simulink model "LH2Ship_Simulink_Summer"  (R2025a)
settings: Solver=VariableStepAuto  StartTime=0.0  StopTime=3600*24*7  FixedStep=0.1  MaxStep=0.5  MinStep=0.001  RelTol=1e-7  AbsTol=1e-7
values from neighbouring files (symbols this model uses):
  BoilerEff = 0.85    [PEMFC_Model.m]
  H2Consumption_kg = H2SupplyMolRate(:,1:iPmaxtot).*H2_kg_mol    [PEMFC_Model.m]
  H2Exhaust_kg = H2ExhaustMolRate(:,1:iPmaxtot).*H2_kg_mol    [PEMFC_Model.m]
  H2hhv = 141.7*10^6    (= 141700000)    [PEMFC_Model.m]
  H2lhv = 119.96*10^6    (= 119960000)    [PEMFC_Model.m]
  H2u = (0.05:0.1:0.95)    [PEMFC_Model.m]
  HeatStorageCapacity = 4.5e10    (= 45000000000)    [PEMFC_Model.m]
  HeatStorageEff = 0.9    [PEMFC_Model.m]
  HeatStorageIC = 1    [PEMFC_Model.m]
  i_FC = iCell(1,1:iPmaxtot)    [PEMFC_Model.m]
  Nstacks = 330    [PEMFC_Model.m]
  PowerElectronicsEff = 0.9    [PEMFC_Model.m]
  RecoveredHeat = NetHeatOut(:,1:iPmaxtot)    [PEMFC_Model.m]
  V_FC = Vout(:,1:iPmaxtot)    [PEMFC_Model.m]
undefined symbols (not defined in the file or in its folder): BatteryCapacity, BattInitialSOC, LH2ColdRecovery_Efficiency, LH2ColdRecovery_EnthalpyGain, mass, Rt, v, VDCBus
libraries: fl_lib x16, nesl_utility x15, simulink x5, slpidlib x2, batteryecm_lib x1, ee_lib x1
(part 1 of 2)
settings Model: Creator=age  LastModifiedBy=alber
settings SolverCC: InitialStep=0.001  MaxConsecutiveMinStep=2  ZeroCrossControl=DisableAll  AlgebraicLoopSolver=TrustRegion
settings DataIOCC: LimitDataPoints=on  MaxDataPoints=10000  ReturnWorkspaceOutputs=off
settings OptimizationCC: LifeSpan=inf
settings DebuggingCC: UnconnectedInputMsg=warning  UnconnectedOutputMsg=warning  UnconnectedLineMsg=warning  AllowSymbolicDim=off  SFUnexpectedBacktrackingDiag=warning  SFNoUnconditionalDefaultTransitionDiag=warning  SFExecutionAtInitializationDiag=none  ArithmeticOperatorsInVariantConditions=warning
settings ModelReferenceCC: EnableRefExpFcnMdlSchedulingChecks=on
settings SFSimCC: SimUseLocalCustomCode=off  CustomCodeUndefinedFunction=UseInterfaceOnly
settings RTWCC: RTWUseLocalCustomCode=off  GPUComputeCapability=3.5
settings CodeAppCC: StateflowObjectComments=on
settings GRTTargetCC: TargetLangStandard=C89/C90 (ANSI)
settings ConfigComp: CovMetricSettings=dw  CovSaveCumulativeToWorkspaceVar=on  CovSaveSingleToWorkspaceVar=on  CovExternalEMLEnable=off  CovSFcnEnable=off
settings SimscapeCC: SimscapeLogLimitData=off  SimscapeLogDataHistory=10000.0

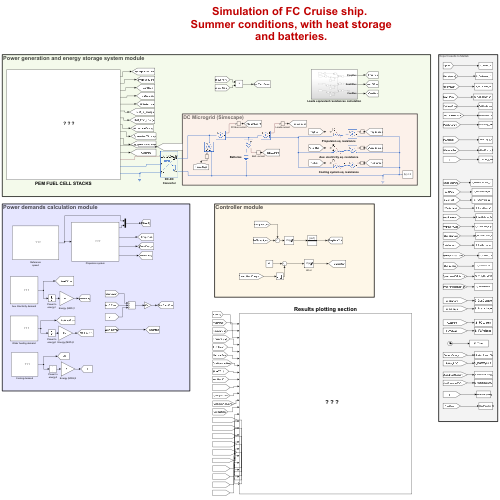
[thumbnail: Simulink's stored preview of the top-level diagram]
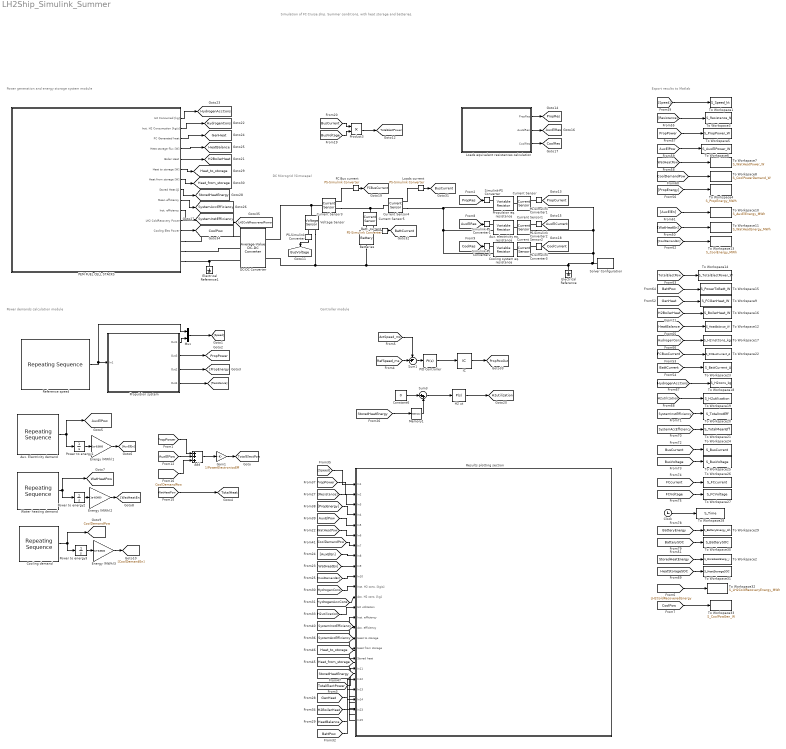
== system LH2Ship_Simulink_Summer ==
  note: Power demands calculation module
  note: Export results to Matlab
  note: Simulation of FC Cruise ship.
      | Summer conditions, with heat storage and batteries.
  note: Power generation and energy storage system module
  note: DC Microgrid (Simscape)
  note: Controller module
  Add : Sum  Inputs=+++
  Aux. Electricity demand : simulink/Sources/Repeating Sequence  rep_seq_t=AuxElectProfile.t  rep_seq_y=AuxElectProfile.Elect  mask(Repeating table){}
      mask Display: image('Aux electricity summer_icon.JPG');
  Aux. electricity eq. resistance : fl_lib/Electrical/Electrical Elements/Variable Resistor  Rmin=2.8571e-4 Ohm  thermalEnable=false  thermal_mass=1 J/K  i_specify=off  i_priority=None  i=0 A  i_nominal_specify=off  i_nominal_value=1  i_nominal_unit=A  v_specify=off  v_priority=None  v=0 V  v_nominal_specify=off  v_nominal_value=1  v_nominal_unit=V  T_specify=off  T_priority=None  T=300 K  T_nominal_specify=off  T_nominal_value=1  T_nominal_unit=K
  Batt. current : nesl_utility/PS-Simulink Converter  PhysicalDomain=network_engine_domain  SubClassName=ps_output  LeftPortType=input  RightPortType=output  PseudoPeriodic=off  Frequencies=[]  VectorFormat=1-D array  Unit=1  AffineConversion=off
  Batteries : batteryecm_lib/Battery  Vnom=100 V  prm_dir=simscape.enum.battery.prm_dir.disabled  R1_dis=2 Ohm  R1_ch=2 Ohm  R1=0.00016667 Ohm  prm_AH=1  AH=6000 hr*A  V1=75 V  AH1=5426.087 hr*A  prm_R2=1  R2=2000 Ohm  Tmeas=298.15 K  charge_measurement_port=simscape.enum.battery.enable.no  prm_dyn=1  Rp1=0.0005 Ohm  tau1=10 s  Rp2=0.005 Ohm  tau2=30 s  Rp3=0.005 Ohm  tau3=30 s  Rp4=0.005 Ohm  tau4=30 s  Rp5=0.005 Ohm  tau5=30 s  prm_fade=1  N_fade=100  AH_fade=45 hr*A  R1_fade=2.02 Ohm  R1_ch_fade=2.02 Ohm  V1_fade=10.35 V  prm_age=simscape.enum.battery.prm_age.disabled  prm_age_OCV=simscape.enum.battery.prm_age_OCV.OCV  OCV_age=0.9  SOC_age=60  Tmeas_age=298.15 K  delta_time_age_vec=[0] d  temperature_age_vec=[273] K  OCV_scaling_age=2.2134e6  OCV_offset_age=1.632e6  temp_exp_age=0.515833569 V  t_exp_age=0.75  Vnom_T2=12 V  R1_T2=2.2 Ohm  R1_T2_dis=2.2 Ohm  R1_T2_ch=2.2 Ohm  V1_T2=11.4 V  R2_T2=2200 Ohm  Rp1_T2=0.005 Ohm  tau1_T2=30 s  Rp2_T2=0.005 Ohm  tau2_T2=30 s  Rp3_T2=0.005 Ohm  tau3_T2=30 s  Rp4_T2=0.005 Ohm  tau4_T2=30 s  Rp5_T2=0.005 Ohm  tau5_T2=30 s  Tmeas2=273.15 K  thermal_port=simscape.enum.thermaleffects.omit  thermal_mass=30000 J/K  i_specify=on  i_priority=Low  i=0 A  i_nominal_specify=off  i_nominal_value=1  i_nominal_unit=A  v_specify=on  v_priority=None  v=100 V  v_nominal_specify=off  v_nominal_value=1  v_nominal_unit=V  charge_specify=on  charge_priority=High  charge=3000 hr*A  charge_nominal_specify=off  charge_nominal_value=1  charge_nominal_unit=hr*A  num_cycles_specify=on  num_cycles_priority=None  num_cycles=0  num_cycles_nominal_specify=off  num_cycles_nominal_value=1  num_cycles_nominal_unit=1  temperature_specify=off  temperature_priority=High  temperature=298.15 K  temperature_nominal_specify=off  temperature_nominal_value=1  temperature_nominal_unit=K
  Clock : Clock
  Constant6 : Constant  Value=0
  Cooling demand : simulink/Sources/Repeating Sequence  rep_seq_t=SpaceCoolingProfile_Summer.t  rep_seq_y=SpaceCoolingProfile_Summer.Cooling  mask(Repeating table){}
      mask Display: image('Cooling demand summer_icon.JPG');
  Cooling system eq. resistance : fl_lib/Electrical/Electrical Elements/Variable Resistor  Rmin=2.8571e-4 Ohm  thermalEnable=false  thermal_mass=1 J/K  i_specify=off  i_priority=None  i=0 A  i_nominal_specify=off  i_nominal_value=1  i_nominal_unit=A  v_specify=off  v_priority=None  v=0 V  v_nominal_specify=off  v_nominal_value=1  v_nominal_unit=V  T_specify=off  T_priority=None  T=300 K  T_nominal_specify=off  T_nominal_value=1  T_nominal_unit=K
  Current Sensor{,1..5} (6 alike) : fl_lib/Electrical/Electrical Sensors/Current Sensor
  DC-DC Converter : ee_lib/Semiconductors & Converters/Converters/Average-Value DC-DC Converter  implementation_option=ee.enum.converters.implementation.behavioral  converter_type=3  control_option=ee.enum.converters.controlinput.dutycycle  efficiency_option=ee.enum.converters.efficiency.constant  efficiency_fixed=100  i_vec=[0, 2, 5] A  efficiency_vec=[90, 95, 98]  Lf=1e-6 H  Rl=0 Ohm  Cf=1e-7 F  Rc=1e-6 Ohm  iL_specify=off  iL_priority=High  iL=0 A  iL_nominal_specify=off  iL_nominal_value=1  iL_nominal_unit=A  vc_specify=off  vc_priority=High  vc=0 V  vc_nominal_specify=off  vc_nominal_value=1  vc_nominal_unit=V
      settings: InternalSimscapePortConfiguration="{\"Bottom\":[],\"Left\":[{\"id\":\"DutyCycle\",\"label\":\"DutyCycle\",\"type\":\"input\"},{\"id\":\"p1\",\"label\":\"1+\",\"type\":\"foundation.electrical.electrical\"},{\"id\":\"n1\",\"label\":\"1-\",\"type\":\"foundation.electrical.electrical\"}],\"Right\":[{\"id\":\"p2\",\"label\":\"2+\",\"type\":\"foundation.electrical.electrical\"},{\"id\":\"n2\",\"label\":\"2-\",\"type\":\"foundation.electrical.electrical\"}],\"Top\":[]}"
  Electrical Reference : fl_lib/Electrical/Electrical Elements/Electrical Reference
  Electrical Reference1 : fl_lib/Electrical/Electrical Elements/Electrical Reference
  Energy (MWh)1 : Gain  Gain=1e-6/3600
  Energy (MWh)2 : Gain  Gain=1e-6/3600
  Energy (MWh)3 : Gain  Gain=1e-6/3600
  FC Bus current : nesl_utility/PS-Simulink Converter  PhysicalDomain=network_engine_domain  SubClassName=ps_output  LeftPortType=input  RightPortType=output  PseudoPeriodic=off  Frequencies=[]  VectorFormat=1-D array  Unit=1  AffineConversion=off
  Gain1 : Gain  Gain=1/PowerElectronicsEff
  H2 ut : slpidlib/PID Controller  Controller=P  Form=Parallel  TimeDomain=Continuous-time  UseExternalTs=off  SampleTime=-1  IntegratorMethod=Forward Euler  FilterMethod=Forward Euler  ControllerParametersSource=internal  P=2.73467181561609e-9  I=5.74544625203428e-08  UseKiTs=off  D=7000000  UseExternalDerivativeSource=off  N=0.01  UseFilter=on  TunerSelectOption=Transfer Function Based (PID Tuner App)  ZeroCross=off  InitialConditionSource=internal  InitialConditionForIntegrator=0.95  InitialConditionForFilter=0.1  DifferentiatorICPrevScaledInput=0  ExternalReset=none  TrackingMode=off  Kt=1  LimitOutput=on  SatLimitsSource=internal  UpperSaturationLimit=0.95  LowerSaturationLimit=0.05  LinearizeAsGain=off  AntiWindupMode=clamping  Kb=1  LimitIntegrator=off  UpperIntegratorSaturationLimit=inf  LowerIntegratorSaturationLimit=-inf  POutMin=[]  POutMax=[]  IOutMin=[]  IOutMax=[]  DOutMin=[]  DOutMax=[]  NOutMin=[]  NOutMax=[]  SumOutMin=[]  SumOutMax=[]  SaturationOutMin=[]  SaturationOutMax=[]  PParamMin=[]  PParamMax=[]  IParamMin=[]  IParamMax=[]  DParamMin=[]  DParamMax=[]  NParamMin=[]  NParamMax=[]  KbParamMin=[]  KbParamMax=[]  KtParamMin=[]  KtParamMax=[]  KbOutMin=[]  KbOutMax=[]  KtOutMin=[]  KtOutMax=[]  IntegratorOutMin=[]  IntegratorOutMax=[]  FilterOutMin=[]  FilterOutMax=[]  SumI1OutMin=[]  SumI1OutMax=[]  SumI2OutMin=[]  SumI2OutMax=[]  SumI3OutMin=[]  SumI3OutMax=[]  SumI4OutMin=[]  SumI4OutMax=[]  SumDOutMin=[]  SumDOutMax=[]  DifferentiatorOutMin=[]  DifferentiatorOutMax=[]  FilterDiffOutCoefMin=[]  FilterDiffOutCoefMax=[]  ReciprocalOutMin=[]  ReciprocalOutMax=[]  SumDenOutMin=[]  SumDenOutMax=[]  SumNumOutMin=[]  SumNumOutMax=[]  DivideOutMin=[]  DivideOutMax=[]  UdiffTsProdOutMin=[]  UdiffTsProdOutMax=[]  NTsProdOutMin=[]  NTsProdOutMax=[]  UintegralTsProdOutMin=[]  UintegralTsProdOutMax=[]  UngainTsProdOutMin=[]  UngainTsProdOutMax=[]  ClampingZeroOutDataTypeStr=Inherit: Inherit via back propagation  ClampingZeroOutMin=[]  ClampingZeroOutMax=[]  FilterDenConstantOutDataTypeStr=Inherit: Inherit via back propagation  FilterDenConstantOutMin=[]  FilterDenConstantOutMax=[]  PCopyOutDataTypeStr=Inherit: Inherit via back propagation  PCopyOutMin=[]  PCopyOutMax=[]  NCopyOutDataTypeStr=Inherit: Inherit via back propagation  NCopyOutMin=[]  NCopyOutMax=[]  IntegratorContinuousStateAttributes=''  IntegratorStateMustResolveToSignalObject=off  IntegratorRTWStateStorageClass=Auto  FilterContinuousStateAttributes=''  FilterStateMustResolveToSignalObject=off  FilterRTWStateStorageClass=Auto  ParallelPVariant=InternalParameters  IdealPVariant=Disabled  IVariant=Disabled  DVariant=Disabled  IntegratorVariant=Disabled  SatVariant=Enabled  AWVariant=Disabled  PCopyVariant=Disabled  TRVariant=Disabled  FdbkBlocksVariant=Forward  IdealPFdbkVariant=Disabled  SatFdbkVariant=Disabled  DerivativeFilterVariant=Disabled  NVariant=Disabled  NCopyVariant=Disabled_SignalSpec  FilterICVariant=Disabled  IntegratorICVariant=Disabled  ExternalResetVariant=Disabled  TRSumVariant=Passthrough  SumFdbkVariant=Disabled  SumVariant=Passthrough_P  TsampFilterVariant=InternalTs  TsampNgainVariant=Passthrough  TsampIntegralVariant=Disabled_SignalSpec  ExternalSaturationOutDataTypeStr=Inherit: Same as second input  DerivativeSourceVariant=Disabled  PreIntVariant=InternalPreInt
  IC : InitialCondition  Value=2e7
  Loads current : nesl_utility/PS-Simulink Converter  PhysicalDomain=network_engine_domain  SubClassName=ps_output  LeftPortType=input  RightPortType=output  PseudoPeriodic=off  Frequencies=[]  VectorFormat=1-D array  Unit=1  AffineConversion=off
  Loads equivalent resistances calculation : Subsystem
  Memory1 : Memory  InitialCondition=HeatStorageIC*HeatStorageCapacity
  Mux : Mux  Inputs=2
  PEM FUEL CELL STACKS : Subsystem
      mask Display: image('Fuel cell_PEM_icon.JPG');
  PID Controller : slpidlib/PID Controller  Controller=PI  Form=Parallel  TimeDomain=Continuous-time  UseExternalTs=off  SampleTime=-1  IntegratorMethod=Forward Euler  FilterMethod=Forward Euler  ControllerParametersSource=internal  P=9967066.66982428  I=15836.3521855852  UseKiTs=off  D=676782585.714132  UseExternalDerivativeSource=off  N=0.00702265439594147  UseFilter=on  TunerSelectOption=Transfer Function Based (PID Tuner App)  InitialConditionSource=internal  InitialConditionForIntegrator=2e7  InitialConditionForFilter=0  DifferentiatorICPrevScaledInput=0  ExternalReset=none  TrackingMode=off  Kt=1  LimitOutput=on  SatLimitsSource=internal  UpperSaturationLimit=60000000  LowerSaturationLimit=-60000000  LinearizeAsGain=off  AntiWindupMode=clamping  Kb=1  LimitIntegrator=off  UpperIntegratorSaturationLimit=inf  LowerIntegratorSaturationLimit=-inf  POutMin=[]  POutMax=[]  IOutMin=[]  IOutMax=[]  DOutMin=[]  DOutMax=[]  NOutMin=[]  NOutMax=[]  SumOutMin=[]  SumOutMax=[]  SaturationOutMin=[]  SaturationOutMax=[]  PParamMin=[]  PParamMax=[]  IParamMin=[]  IParamMax=[]  DParamMin=[]  DParamMax=[]  NParamMin=[]  NParamMax=[]  KbParamMin=[]  KbParamMax=[]  KtParamMin=[]  KtParamMax=[]  KbOutMin=[]  KbOutMax=[]  KtOutMin=[]  KtOutMax=[]  IntegratorOutMin=[]  IntegratorOutMax=[]  FilterOutMin=[]  FilterOutMax=[]  SumI1OutMin=[]  SumI1OutMax=[]  SumI2OutMin=[]  SumI2OutMax=[]  SumI3OutMin=[]  SumI3OutMax=[]  SumI4OutMin=[]  SumI4OutMax=[]  SumDOutMin=[]  SumDOutMax=[]  DifferentiatorOutMin=[]  DifferentiatorOutMax=[]  FilterDiffOutCoefMin=[]  FilterDiffOutCoefMax=[]  ReciprocalOutMin=[]  ReciprocalOutMax=[]  SumDenOutMin=[]  SumDenOutMax=[]  SumNumOutMin=[]  SumNumOutMax=[]  DivideOutMin=[]  DivideOutMax=[]  UdiffTsProdOutMin=[]  UdiffTsProdOutMax=[]  NTsProdOutMin=[]  NTsProdOutMax=[]  UintegralTsProdOutMin=[]  UintegralTsProdOutMax=[]  UngainTsProdOutMin=[]  UngainTsProdOutMax=[]  ClampingZeroOutDataTypeStr=Inherit: Inherit via back propagation  ClampingZeroOutMin=[]  ClampingZeroOutMax=[]  FilterDenConstantOutDataTypeStr=Inherit: Inherit via back propagation  FilterDenConstantOutMin=[]  FilterDenConstantOutMax=[]  PCopyOutDataTypeStr=Inherit: Inherit via back propagation  PCopyOutMin=[]  PCopyOutMax=[]  NCopyOutDataTypeStr=Inherit: Inherit via back propagation  NCopyOutMin=[]  NCopyOutMax=[]  IntegratorContinuousStateAttributes=''  IntegratorStateMustResolveToSignalObject=off  IntegratorRTWStateStorageClass=Auto  FilterContinuousStateAttributes=''  FilterStateMustResolveToSignalObject=off  FilterRTWStateStorageClass=Auto  ParallelPVariant=InternalParameters  IdealPVariant=Disabled  IVariant=InternalParameters  DVariant=Disabled  IntegratorVariant=Continuous  SatVariant=Enabled  AWVariant=ContClampingParallel  PCopyVariant=Disabled  TRVariant=Disabled  FdbkBlocksVariant=Forward  IdealPFdbkVariant=Disabled  SatFdbkVariant=Disabled  DerivativeFilterVariant=Disabled  NVariant=Disabled  NCopyVariant=Disabled_SignalSpec  FilterICVariant=Disabled  IntegratorICVariant=InternalICs  ExternalResetVariant=Disabled  TRSumVariant=Passthrough  SumFdbkVariant=Disabled  SumVariant=Sum_PI  TsampFilterVariant=InternalTs  TsampNgainVariant=Passthrough  TsampIntegralVariant=Disabled_SignalSpec  ExternalSaturationOutDataTypeStr=Inherit: Same as second input  DerivativeSourceVariant=Disabled  PreIntVariant=InternalPreInt
  PS-Simulink Converter{,1..3} (4 alike) : nesl_utility/PS-Simulink Converter  PhysicalDomain=network_engine_domain  SubClassName=ps_output  LeftPortType=input  RightPortType=output  PseudoPeriodic=off  Frequencies=[]  VectorFormat=1-D array  Unit=1  AffineConversion=off
  Power to energy1 : Integrator  LowerSaturationLimit=0
  Power to energy2 : Integrator  LowerSaturationLimit=0
  Power to energy3 : Integrator  LowerSaturationLimit=0
  Product3 : Product
  Propulsion eq. resistance : fl_lib/Electrical/Electrical Elements/Variable Resistor  Rmin=2.8571e-4 Ohm  thermalEnable=false  thermal_mass=1 J/K  i_specify=off  i_priority=None  i=0 A  i_nominal_specify=off  i_nominal_value=1  i_nominal_unit=A  v_specify=off  v_priority=None  v=0 V  v_nominal_specify=off  v_nominal_value=1  v_nominal_unit=V  T_specify=off  T_priority=None  T=300 K  T_nominal_specify=off  T_nominal_value=1  T_nominal_unit=K
  Propulsion system : Subsystem
      mask Display: image('Propusion engine.jpg');
  Reference speed : simulink/Sources/Repeating Sequence  rep_seq_t=SpeedProfile.Time  rep_seq_y=SpeedProfile.Speed  mask(Repeating table){}
      mask Display: image('RefSpeed_icon.PNG');
  Results plotting section : Subsystem
      mask Display: image('222-2224981_data-visualization-icon-circle.png.jpg');
  Simulink-PS Converter : nesl_utility/Simulink-PS Converter  PhysicalDomain=network_engine_domain  SubClassName=ps_input  LeftPortType=input  RightPortType=output  PseudoPeriodic=off  Frequencies=[]  NoiseDistribution=none  NoiseParameters=[]  Unit=1  AffineConversion=off  FilteringAndDerivatives=provide  SimscapeFilterOrder=1  InputFilterTimeConstant=0.001  UdotUserProvided=0
  Simulink-PS Converter1 : nesl_utility/Simulink-PS Converter  PhysicalDomain=network_engine_domain  SubClassName=ps_input  LeftPortType=input  RightPortType=output  PseudoPeriodic=off  Frequencies=[]  NoiseDistribution=none  NoiseParameters=[]  Unit=1  AffineConversion=off  FilteringAndDerivatives=provide  SimscapeFilterOrder=1  InputFilterTimeConstant=0.001  UdotUserProvided=0
  Simulink-PS Converter2 : nesl_utility/Simulink-PS Converter  PhysicalDomain=network_engine_domain  SubClassName=ps_input  LeftPortType=input  RightPortType=output  PseudoPeriodic=off  Frequencies=[]  NoiseDistribution=none  NoiseParameters=[]  Unit=1  AffineConversion=off  FilteringAndDerivatives=provide  SimscapeFilterOrder=1  InputFilterTimeConstant=0.001  UdotUserProvided=0
  Solver Configuration : nesl_utility/Solver Configuration  PhysicalDomain=network_engine_domain  SubClassName=solver  LeftPortType=input  RightPortType=generic  Tones=[]  Harmonics=[]  SimulateNoise=off  Profile=off  UseLocalSampling=off  EnableSwitchedLinearOptims=on  FrequencyDomain=off  UseCCode=off  RelTol=0.001  AbsTol=1e-06  MinStep=1e-09  ToWorkspace=off  RevertToSquareIcSolve=off  NumHomotopyIterations=100  PhasorMode=off  PhasorModeNumHarmonics=1  ConsistencySolver=NEWTON_FTOL  IndexReductionMethod=DerivativeReplacement  DoDC=on  ResidualTolerance=1e-09  ConsistencyTolSource=GLOBAL  ConsistencyAbsTol=0.001  ConsistencyRelTol=0.001  ConsistencyTolFactor=0.001  UseLocalSolver=off  LocalSolverChoice=NE_BACKWARD_EULER_ADVANCER  ResolveIndetEquations=on  FunctionEvalNumThread=1  LocalSolverSampleTime=0.001  DoFixedCost=off  MaxNonlinIter=3  MaxModeIter=2  ComputeImpulses=off  ImpulseIterations=2  LinearAlgebra=auto  LinearAlgebraNumThread=0  EquationFormulation=NE_TIME_EF  DelaysMemoryBudget=1024  AutomaticFiltering=on  FilteringTimeConstant=0.001  PartitionStorageMethod=AS_NEEDED  PartitionMemoryBudget=1024  PartitionMethod=FAST  MultibodyUseLocalSolver=off  MultibodyLocalSolverChoice=ODE1  MultibodyLocalSolverSampleTime=0.001
  Sum1 : Sum  Inputs=-+|
  Sum3 : Sum  Inputs=|++
  To Workspace1 : ToWorkspace  VariableName=S_Speed_kt  SampleTime=30
  To Workspace10 : ToWorkspace  VariableName=S_AuxElEnergy_MWh  SampleTime=30
  To Workspace11 : ToWorkspace  VariableName=S_WatHeatEnergy_MWh  SampleTime=30
  To Workspace12 : ToWorkspace  VariableName=S_HeatBalance_W  SampleTime=30
  To Workspace13 : ToWorkspace  VariableName=S_CoolEnergy_MWh  SampleTime=30
  To Workspace14 : ToWorkspace  VariableName=S_TotalElectPower_W  SampleTime=30
  To Workspace15 : ToWorkspace  VariableName=S_PowerToBatt_W  SampleTime=30
  To Workspace16 : ToWorkspace  VariableName=S_BoilerHeat_W  SampleTime=30
  To Workspace17 : ToWorkspace  VariableName=S_H2instCons_kgs  SampleTime=30
  To Workspace18 : ToWorkspace  VariableName=S_H2cons_kg  SampleTime=30
  To Workspace19 : ToWorkspace  VariableName=S_H2utilization  SampleTime=30
  To Workspace2 : ToWorkspace  VariableName=S_StoredHeatEnergy_J  SampleTime=30
  To Workspace20 : ToWorkspace  VariableName=S_TotalInstEff  SampleTime=30
  To Workspace21 : ToWorkspace  VariableName=S_TotalMeanEff  SampleTime=30
  To Workspace22 : ToWorkspace  VariableName=S_FCBusCurrent_A  SampleTime=30
  To Workspace23 : ToWorkspace  VariableName=S_BattCurrent_A  SampleTime=30
  To Workspace24 : ToWorkspace  VariableName=S_BusCurrent  SampleTime=30
  To Workspace25 : ToWorkspace  VariableName=S_BusVoltage  SampleTime=30
  To Workspace26 : ToWorkspace  VariableName=S_FCcurrent  SampleTime=30
  To Workspace27 : ToWorkspace  VariableName=S_FCVoltage  SampleTime=30
  To Workspace28 : ToWorkspace  VariableName=S_Time  SampleTime=30
  To Workspace29 : ToWorkspace  VariableName=S_BatteryEnergy_Ah  SampleTime=30
  To Workspace3 : ToWorkspace  VariableName=S_Resistance_N  SampleTime=30
  To Workspace30 : ToWorkspace  VariableName=S_BatterySOC  SampleTime=30
  To Workspace31 : ToWorkspace  VariableName=S_HeatStorageSOC  SampleTime=30
  To Workspace32 : ToWorkspace  VariableName=S_LH2ColdRecoveryEnergy_MWh  SampleTime=30
  To Workspace33 : ToWorkspace  VariableName=S_CoolPowGen_W  SampleTime=30
  To Workspace4 : ToWorkspace  VariableName=S_PropEnergy_MWh  SampleTime=30
  To Workspace5 : ToWorkspace  VariableName=S_PropPower_W  SampleTime=30
  To Workspace6 : ToWorkspace  VariableName=S_AuxElPower_W  SampleTime=30
  To Workspace7 : ToWorkspace  VariableName=S_WatHeatPower_W  SampleTime=30
  To Workspace8 : ToWorkspace  VariableName=S_CoolPowerDemand_W  SampleTime=30
  To Workspace9 : ToWorkspace  VariableName=S_FCGenHeat_W  SampleTime=30
  Voltage Sensor : fl_lib/Electrical/Electrical Sensors/Voltage Sensor
  Water heating demand : simulink/Sources/Repeating Sequence  rep_seq_t=WaterHeatingProfile.t  rep_seq_y=WaterHeatingProfile.Heat  mask(Repeating table){}
      mask Display: image('Hot water summer_icon.JPG');
  tag scope: AuxElCurrent=global, AuxElPow=global, AuxElRes=global, BattCurrent=global, BusCurrent=global, BusVoltage=global, CoolCurrent=global, CoolDemandPow=global, CoolPow=global, CoolRes=global, FCBusCurrent=global, GenHeat=global, H2BoilerHeat=global, H2utilization=global, HeatBalance=global, Heat_from_storage=global, Heat_to_storage=global, HydrogenAccCons=global, HydrogenCons=global, LH2ColdRecoveredPower=global, PropCurrent=global, PropPowOut=global, PropPower=global, PropRes=global, StoredHeatEnergy=global, SystemAccEfficiency=global, SystemInstEfficiency=global, TotalElectPow=global, TotalElectPower=global, TotalHeat=global, WatHeatPow=global
  wires:
  Power to energy1/1 -> Energy (MWh)1/1
  Power to energy3/1 -> Energy (MWh)3/1
  Propulsion system/4(Out4) -> [Resistance]
  Water heating demand/1 -> [WatHeatPow], Power to energy2/1
  Mux/1 -> [Speed]
  Propulsion system/3(Out2) -> [PropEnergy]
  Power to energy2/1 -> Energy (MWh)2/1
  [CoolDemandPow] -> Add/3
  Cooling demand/1 -> [CoolDemandPow], Power to energy3/1
  [WatHeatPow] -> [TotalHeat]
  [PropPower] -> Add/1
  [AuxElPow] -> Add/2
  Propulsion system/1(Out1) -> Mux/2
  Reference speed/1 -> Mux/1, Propulsion system/1(In1)
  Energy (MWh)3/1 -> [CoolDemandEn]
  Energy (MWh)2/1 -> [WatHeatEn]
  Add/1 -> Gain1/1
  Aux. Electricity demand/1 -> [AuxElPow], Power to energy1/1
  Energy (MWh)1/1 -> [AuxElEn]
  PS-Simulink Converter/1 -> [BusVoltage]
  PS-Simulink Converter1/1 -> [PropCurrent]
  Loads equivalent resistances calculation/1(PropRes) -> [PropRes]
  [PropRes] -> Simulink-PS Converter/1
  [AuxElRes] -> Simulink-PS Converter1/1
  PS-Simulink Converter2/1 -> [AuxElCurrent]
  Loads equivalent resistances calculation/2(AuxElRes) -> [AuxElRes]
  Loads equivalent resistances calculation/3(CoolRes) -> [CoolRes]
  PS-Simulink Converter3/1 -> [CoolCurrent]
  [CoolRes] -> Simulink-PS Converter2/1
  FC Bus current/1 -> [FCBusCurrent]
  PEM FUEL CELL STACKS/7(Heat from storage [W]) -> [Heat_from_storage]
  PEM FUEL CELL STACKS/8(Stored Heat [J]) -> [StoredHeatEnergy]
  PEM FUEL CELL STACKS/6(Heat to storage [W]) -> [Heat_to_storage]
  PEM FUEL CELL STACKS/5(Boiler Heat) -> [H2BoilerHeat]
  PEM FUEL CELL STACKS/4(Heat storage flux [W]) -> [HeatBalance]
  PEM FUEL CELL STACKS/3(FC Generated heat) -> [GenHeat]
  PEM FUEL CELL STACKS/2(Inst. H2 Consumption [kg/s]) -> [HydrogenCons]
  PEM FUEL CELL STACKS/1(H2 Consumed [kg]) -> [HydrogenAccCons]
  [Speed] -> Results plotting section/1(In1)
  [BattPow] -> Results plotting section/23(In23)
  [GenHeat] -> Results plotting section/20(In12)
  [WatHeatEn] -> Results plotting section/9(In9)
  [Heat_to_storage] -> Results plotting section/16(Heat to storage)
  [SystemAccEfficiency] -> Results plotting section/15(Acc. efficiency)
  [H2utilization] -> Results plotting section/13(H2 utilization)
  [CoolDemandPow] -> Results plotting section/7(In7)
  [AuxElPow] -> Results plotting section/5(In5)
  [StoredHeatEnergy] -> Results plotting section/18(Stored heat)
  [SystemInstEfficiency] -> Results plotting section/14(Inst. efficiency)
  [AuxElEn] -> Results plotting section/8(In8)
  [Heat_from_storage] -> Results plotting section/17(Heat from storage)
  [HydrogenCons] -> Results plotting section/11(Inst. H2 cons. [kg/s])
  [HeatBalance] -> Results plotting section/22(In14)
  [PropPower] -> Results plotting section/2(In2)
  [PropEnergy] -> Results plotting section/4(In4)
  [HydrogenAccCons] -> Results plotting section/12(Acc. H2 cons. [kg])
  [H2BoilerHeat] -> Results plotting section/21(In13)
  [Resistance] -> Results plotting section/3(In3)
  [WatHeatPow] -> Results plotting section/6(In6)
  [CoolDemandEn] -> Results plotting section/10(In10)
  PEM FUEL CELL STACKS/9(Mean efficiency) -> [SystemAccEfficiency]
  PEM FUEL CELL STACKS/10(Inst. efficiency) -> [SystemInstEfficiency]
  Loads current/1 -> [BusCurrent]
  Batt. current/1 -> [BattCurrent]
  [WatHeatEn] -> To Workspace11/1
  [Resistance] -> To Workspace3/1
  [GenHeat] -> To Workspace9/1
  [Speed] -> To Workspace1/1
  [SystemAccEfficiency] -> To Workspace21/1
  [WatHeatPow] -> To Workspace7/1
  [PropPower] -> To Workspace5/1
  [HydrogenCons] -> To Workspace17/1
  [FCBusCurrent] -> To Workspace22/1
  [BattPow] -> To Workspace15/1
  [BattCurrent] -> To Workspace23/1
  [SystemInstEfficiency] -> To Workspace20/1
  [HydrogenAccCons] -> To Workspace18/1
  [H2utilization] -> To Workspace19/1
  [PropEnergy] -> To Workspace4/1
  [H2BoilerHeat] -> To Workspace16/1
  [HeatBalance] -> To Workspace12/1
  [CoolDemandPow] -> To Workspace8/1
  [AuxElPow] -> To Workspace6/1
  [CoolDemandEn] -> To Workspace13/1
  [AuxElEn] -> To Workspace10/1
  [TotalElectPow] -> To Workspace14/1
  [BusCurrent] -> To Workspace24/1
  [BusVoltage] -> To Workspace25/1
  [FCcurrent] -> To Workspace26/1
  [FCVoltage] -> To Workspace27/1
  Clock/1 -> To Workspace28/1
  [BatterySOC] -> To Workspace30/1
  [BatteryEnergy] -> To Workspace29/1
  Propulsion system/2(Out3) -> [PropPower]
  [HeatStorageSOC] -> To Workspace31/1
  [StoredHeatEnergy] -> To Workspace2/1
  Product3/1 -> [TotalElectPower]
  [BusVoltage] -> Product3/2
  [BusCurrent] -> Product3/1
  [TotalElectPower] -> Results plotting section/19(In11)
  Sum3/1 -> H2 ut/1
  [StoredHeatEnergy] -> Memory1/1
  H2 ut/1 -> [H2utilization]
  Constant6/1 -> Sum3/1
  Memory1/1 -> Sum3/2
  Sum1/1 -> PID Controller/1
  PID Controller/1 -> IC/1
  IC/1 -> [PropPowOut]
  [RefSpeed_ms] -> Sum1/2
  [ActSpeed_ms] -> Sum1/1
  Gain1/1 -> [TotalElectPow]
  PEM FUEL CELL STACKS/12(Cooling Elec Power) -> [CoolPow]
  PEM FUEL CELL STACKS/11(LH2 ColdRecovery Power) -> [LH2ColdRecoveredPower]
  [LH2ColdRecoveredEnergy] -> To Workspace32/1
  [CoolPow] -> To Workspace33/1
  connections:
  Simulink-PS Converter/RConn1 -- Propulsion eq. resistance/LConn1
  Current Sensor/LConn1 -- Propulsion eq. resistance/RConn1
  Current Sensor/RConn2 -- Current Sensor1/RConn2 -- Current Sensor2/RConn2 -- Voltage Sensor/RConn2 -- DC-DC Converter/RConn2 -- Batteries/RConn1 -- Electrical Reference/LConn1 -- Solver Configuration/RConn1
  PS-Simulink Converter/LConn1 -- Voltage Sensor/RConn1
  Current Sensor/RConn1 -- PS-Simulink Converter1/LConn1
  Aux. electricity eq. resistance/LConn2 -- Cooling system eq. resistance/LConn2 -- Current Sensor4/RConn2 -- Propulsion eq. resistance/LConn2
  PEM FUEL CELL STACKS/RConn1 -- DC-DC Converter/LConn1
  PEM FUEL CELL STACKS/RConn2 -- DC-DC Converter/LConn2
  PEM FUEL CELL STACKS/RConn3 -- DC-DC Converter/LConn3 -- Electrical Reference1/LConn1
  Current Sensor1/LConn1 -- Aux. electricity eq. resistance/RConn1
  Current Sensor1/RConn1 -- PS-Simulink Converter2/LConn1
  Simulink-PS Converter1/RConn1 -- Aux. electricity eq. resistance/LConn1
  Simulink-PS Converter2/RConn1 -- Cooling system eq. resistance/LConn1
  Current Sensor2/RConn1 -- PS-Simulink Converter3/LConn1
  Current Sensor2/LConn1 -- Cooling system eq. resistance/RConn1
  Current Sensor3/RConn1 -- FC Bus current/LConn1
  Voltage Sensor/LConn1 -- Current Sensor3/LConn1 -- DC-DC Converter/RConn1
  Current Sensor3/RConn2 -- Current Sensor5/LConn1 -- Current Sensor4/LConn1
  Current Sensor4/RConn1 -- Loads current/LConn1
  Current Sensor5/RConn1 -- Batt. current/LConn1
  Batteries/LConn1 -- Current Sensor5/RConn2

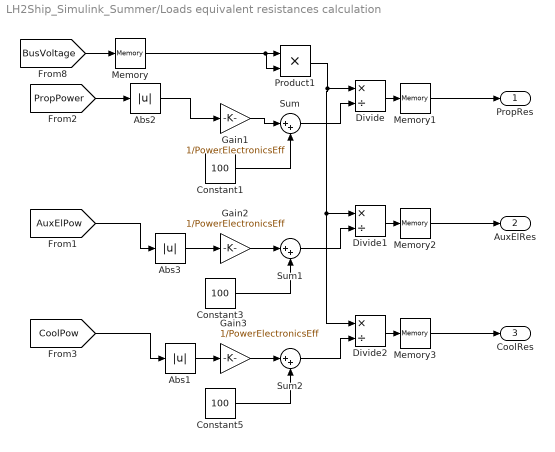
== system LH2Ship_Simulink_Summer/Loads equivalent resistances calculation ==
  Abs1 : Abs  SaturateOnIntegerOverflow=off
  Abs2 : Abs  SaturateOnIntegerOverflow=off
  Abs3 : Abs  SaturateOnIntegerOverflow=off
  Constant1 : Constant  Value=100
  Constant3 : Constant  Value=100
  Constant5 : Constant  Value=100
  Divide : Product  Inputs=*/
  Divide1 : Product  Inputs=*/
  Divide2 : Product  Inputs=*/
  Gain1 : Gain  Gain=1/PowerElectronicsEff
  Gain2 : Gain  Gain=1/PowerElectronicsEff
  Gain3 : Gain  Gain=1/PowerElectronicsEff
  Memory : Memory  InitialCondition=100
  Memory1 : Memory  InitialCondition=0.0005
  Memory2 : Memory  InitialCondition=0.0005
  Memory3 : Memory  InitialCondition=0.001
  Product1 : Product
  Sum : Sum  Inputs=|++
  Sum1 : Sum  Inputs=|++
  Sum2 : Sum  Inputs=|++
  PropRes : Outport  VectorParamsAs1DForOutWhenUnconnected=off
  AuxElRes : Outport  Port=2  VectorParamsAs1DForOutWhenUnconnected=off
  CoolRes : Outport  Port=3  VectorParamsAs1DForOutWhenUnconnected=off
  wires:
  Divide/1 -> Memory1/1
  Memory/1 -> Product1/2, Product1/1
  Constant1/1 -> Sum/2
  [BusVoltage] -> Memory/1
  Sum/1 -> Divide/2
  Memory1/1 -> PropRes/1
  [AuxElPow] -> Abs3/1
  Sum1/1 -> Divide1/2
  Constant3/1 -> Sum1/2
  Divide1/1 -> Memory2/1
  Memory2/1 -> AuxElRes/1
  Product1/1 -> Divide2/1, Divide1/1, Divide/1
  Sum2/1 -> Divide2/2
  [CoolPow] -> Abs1/1
  Constant5/1 -> Sum2/2
  Memory3/1 -> CoolRes/1
  [PropPower] -> Abs2/1
  Divide2/1 -> Memory3/1
  Gain1/1 -> Sum/1
  Abs2/1 -> Gain1/1
  Abs3/1 -> Gain2/1
  Gain2/1 -> Sum1/1
  Abs1/1 -> Gain3/1
  Gain3/1 -> Sum2/1

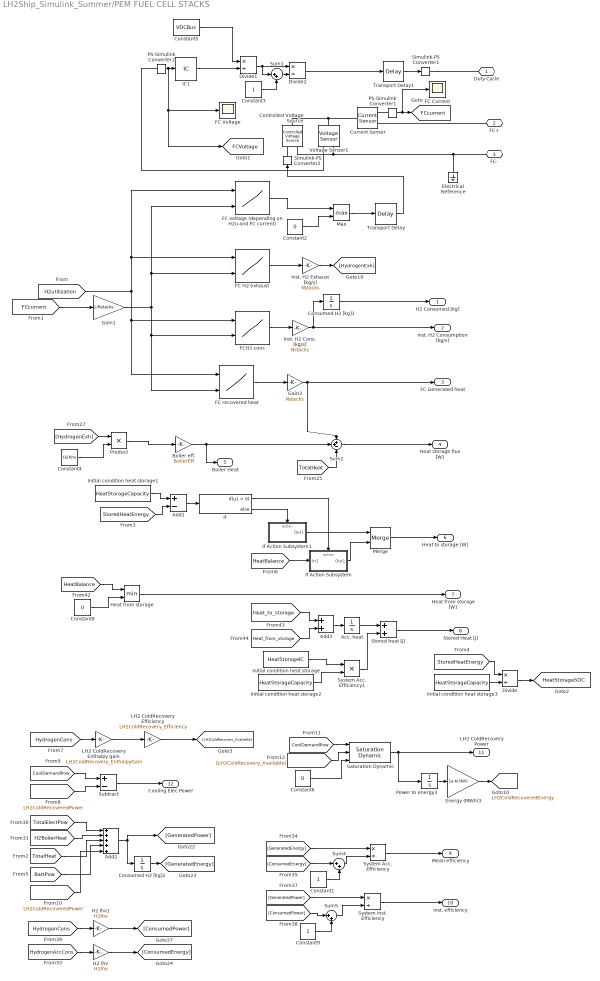
== system LH2Ship_Simulink_Summer/PEM FUEL CELL STACKS ==
  Acc. heat : Integrator
  Add1 : Sum  Inputs=+-
  Add2 : Sum  Inputs=+++++
  Add3 : Sum
  Boiler eff. : Gain  Gain=BoilerEff
  Constant1 : Constant
  Constant2 : Constant  Value=0
  Constant3 : Constant
  Constant4 : Constant  Value=H2hhv
  Constant5 : Constant  Value=VDCBus
  Constant6 : Constant  Value=0
  Constant8 : Constant  Value=0
  Constant9 : Constant
  Consumed H2 [kg]1 : Integrator
  Consumed H2 [kg]2 : Integrator
  Controlled Voltage Source : fl_lib/Electrical/Electrical Sources/Controlled Voltage Source
  Current Sensor : fl_lib/Electrical/Electrical Sensors/Current Sensor
  Divide : Product  Inputs=*/
  Divide1 : Product  Inputs=*/
  Divide2 : Product  Inputs=*/
  Electrical Reference : fl_lib/Electrical/Electrical Elements/Electrical Reference
  Energy (MWh)3 : Gain  Gain=1e-6/3600
  FC Current : Scope
      settings: SampleTime=10  ActiveDisplayYMinimum=215810.81022  ActiveDisplayYMaximum=347573.91191  DataLoggingVariableName=ScopeData2  DataLoggingSaveFormat=Array
  FC H2 exhaust : Lookup_n-D  BreakpointsForDimension1=H2u  BreakpointsForDimension2=i_FC  Table=H2Exhaust_kg  InternalRulePriority=Speed  RndMeth=Simplest
      settings: InputPortMap=u0,u1
  FC Voltage : Scope
      settings: SampleTime=10  ActiveDisplayYMinimum=108.78379  ActiveDisplayYMaximum=120.9459  DataLoggingSaveFormat=Array
  FC recovered heat : Lookup_n-D  BreakpointsForDimension1=H2u  BreakpointsForDimension2=i_FC  Table=RecoveredHeat  InternalRulePriority=Speed  RndMeth=Simplest
      settings: InputPortMap=u0,u1
  FC voltage (depending on H2u and FC current) : Lookup_n-D  BreakpointsForDimension1=H2u  BreakpointsForDimension2=i_FC  Table=V_FC  InternalRulePriority=Speed  RndMeth=Simplest
      settings: InputPortMap=u0,u1
  FCH2 cons : Lookup_n-D  BreakpointsForDimension1=H2u  BreakpointsForDimension2=i_FC  Table=H2Consumption_kg  InternalRulePriority=Speed  RndMeth=Simplest
      settings: InputPortMap=u0,u1
  Gain1 : Gain  Gain=1/Nstacks
  Gain3 : Gain  Gain=Nstacks
  H2 lhv : Gain  Gain=H2lhv
  H2 lhv1 : Gain  Gain=H2lhv
  "Heat from storage " : MinMax  Inputs=2
  IC1 : InitialCondition  Value=110
  If : If
  If Action Subsystem : Subsystem  TreatAsAtomicUnit=on
  If Action Subsystem1 : Subsystem  TreatAsAtomicUnit=on
  Initial condition heat storage : Constant  Value=HeatStorageIC
  Initial condition heat storage1 : Constant  Value=HeatStorageCapacity
  Initial condition heat storage2 : Constant  Value=HeatStorageCapacity
  Initial condition heat storage3 : Constant  Value=HeatStorageCapacity
  Inst. H2 Cons. [kg/s] : Gain  Gain=Nstacks
  Inst. H2 Exhaust [kg/s] : Gain  Gain=Nstacks
  LH2 ColdRecovery Efficiency : Gain  Gain=LH2ColdRecovery_Efficiency
  LH2 ColdRecovery Enthalpy gain : Gain  Gain=LH2ColdRecovery_EnthalpyGain
  Max : MinMax  Function=max  Inputs=2
  Merge : Merge
  PS-Simulink Converter1 : nesl_utility/PS-Simulink Converter  PhysicalDomain=network_engine_domain  SubClassName=ps_output  LeftPortType=input  RightPortType=output  PseudoPeriodic=off  Frequencies=[]  VectorFormat=1-D array  Unit=1  AffineConversion=off
  PS-Simulink Converter2 : nesl_utility/PS-Simulink Converter  PhysicalDomain=network_engine_domain  SubClassName=ps_output  LeftPortType=input  RightPortType=output  PseudoPeriodic=off  Frequencies=[]  VectorFormat=1-D array  Unit=1  AffineConversion=off
  Power to energy3 : Integrator  LowerSaturationLimit=0
  Product : Product
  Saturation Dynamic : simulink/Discontinuities/Saturation Dynamic  OutMin=0  OutMax=[]  OutDataTypeStr=Inherit: Same as second input  OutDataType=fixdt(1, 16)  OutScaling=2^-10  DoSatur=off
  Simulink-PS Converter1 : nesl_utility/Simulink-PS Converter  PhysicalDomain=network_engine_domain  SubClassName=ps_input  LeftPortType=input  RightPortType=output  PseudoPeriodic=off  Frequencies=[]  NoiseDistribution=none  NoiseParameters=[]  Unit=1  AffineConversion=off  FilteringAndDerivatives=provide  SimscapeFilterOrder=1  InputFilterTimeConstant=0.001  UdotUserProvided=0
  Simulink-PS Converter2 : nesl_utility/Simulink-PS Converter  PhysicalDomain=network_engine_domain  SubClassName=ps_input  LeftPortType=input  RightPortType=output  PseudoPeriodic=off  Frequencies=[]  NoiseDistribution=none  NoiseParameters=[]  Unit=1  AffineConversion=off  FilteringAndDerivatives=provide  SimscapeFilterOrder=1  InputFilterTimeConstant=0.001  UdotUserProvided=0
  Stored heat [J] : Sum
  Subtract : Sum  Inputs=+-
  Sum1 : Sum  Inputs=|++
  Sum2 : Sum  Inputs=++-
  Sum4 : Sum  Inputs=|++
  Sum5 : Sum  Inputs=|++
  System Acc. Efficiency : Product  Inputs=*/
  System Acc. Efficiency1 : Product  Inputs=**
  System inst. Efficiency : Product  Inputs=*/
  Transport Delay : TransportDelay  DelayTime=60  InitialOutput=110
  Transport Delay1 : TransportDelay  DelayTime=30  InitialOutput=0.4762
  Voltage Sensor1 : fl_lib/Electrical/Electrical Sensors/Voltage Sensor
  Duty Cycle : PMIOPort  Side=Right
  FC+ : PMIOPort  Port=2  Side=Right
  FC- : PMIOPort  Port=3  Side=Right
  H2 Consumed [kg] : Outport  VectorParamsAs1DForOutWhenUnconnected=off
  Inst. H2 Consumption [kg/s] : Outport  Port=2  VectorParamsAs1DForOutWhenUnconnected=off
  FC Generated heat : Outport  Port=3  VectorParamsAs1DForOutWhenUnconnected=off
  Heat storage flux [W] : Outport  Port=4  VectorParamsAs1DForOutWhenUnconnected=off
  Boiler Heat : Outport  Port=5  VectorParamsAs1DForOutWhenUnconnected=off
  Heat to storage [W] : Outport  Port=6  VectorParamsAs1DForOutWhenUnconnected=off
  Heat from storage [W] : Outport  Port=7  VectorParamsAs1DForOutWhenUnconnected=off
  Stored Heat [J] : Outport  Port=8  VectorParamsAs1DForOutWhenUnconnected=off
  Mean efficiency : Outport  Port=9  VectorParamsAs1DForOutWhenUnconnected=off
  Inst. efficiency : Outport  Port=10  VectorParamsAs1DForOutWhenUnconnected=off
  LH2 ColdRecovery Power : Outport  Port=11  VectorParamsAs1DForOutWhenUnconnected=off
  Cooling Elec Power : Outport  Port=12  VectorParamsAs1DForOutWhenUnconnected=off
  tag scope: FCVoltage=global, FCcurrent=global, HeatStorageSOC=global, LH2ColdRecoveredEnergy=global
  wires:
  Constant3/1 -> Sum1/2
  Divide1/1 -> Sum1/1, Divide2/1
  Constant5/1 -> Divide1/1
  PS-Simulink Converter2/1 -> [FCVoltage], FC Voltage/1, IC1/1
  Sum1/1 -> Divide2/2
  FC voltage (depending on H2u and FC current)/1 -> Max/1
  [H2utilization] -> FC recovered heat/1, FCH2 cons/1, FC H2 exhaust/1, FC voltage (depending on H2u and FC current)/1
  Gain1/1 -> FC H2 exhaust/2, FC voltage (depending on H2u and FC current)/2, FCH2 cons/2, FC recovered heat/2
  PS-Simulink Converter1/1 -> FC Current/1, [FCcurrent]
  Constant2/1 -> Max/2
  FC H2 exhaust/1 -> Inst. H2 Exhaust [kg/s]/1
  FCH2 cons/1 -> Inst. H2 Cons. [kg/s]/1
  Constant4/1 -> Product/2
  Sum2/1 -> Heat storage flux [W]/1
  Product/1 -> Boiler eff./1
  Inst. H2 Cons. [kg/s]/1 -> Inst. H2 Consumption [kg/s]/1, Consumed H2 [kg]1/1
  [HydrogenExh] -> Product/1
  Inst. H2 Exhaust [kg/s]/1 -> [HydrogenExh]
  Consumed H2 [kg]1/1 -> H2 Consumed [kg]/1
  Boiler eff./1 -> Boiler Heat/1, Sum2/2
  Gain3/1 -> FC Generated heat/1, Sum2/1
  [TotalHeat] -> Sum2/3
  FC recovered heat/1 -> Gain3/1
  Constant8/1 -> "Heat from storage "/2
  [Heat_to_storage] -> Add3/1
  "Heat from storage "/1 -> Heat from storage [W]/1
  [Heat_from_storage] -> Add3/2
  [HeatBalance] -> "Heat from storage "/1
  Acc. heat/1 -> Stored heat [J]/1
  Add3/1 -> Acc. heat/1
  [BattPow] -> Add2/4
  System Acc. Efficiency/1 -> Mean efficiency/1
  [TotalHeat] -> Add2/3
  [HydrogenAccCons] -> H2 lhv/1
  [TotalElectPow] -> Add2/1
  System inst. Efficiency/1 -> Inst. efficiency/1
  [GeneratedEnergy] -> System Acc. Efficiency/1
  Consumed H2 [kg]2/1 -> [GeneratedEnergy]
  H2 lhv1/1 -> [ConsumedPower]
  H2 lhv/1 -> [ConsumedEnergy]
  [ConsumedEnergy] -> Sum4/1
  [H2BoilerHeat] -> Add2/2
  Add2/1 -> [GeneratedPower], Consumed H2 [kg]2/1
  [HydrogenCons] -> H2 lhv1/1
  [GeneratedPower] -> System inst. Efficiency/1
  [FCcurrent] -> Gain1/1
  Constant1/1 -> Sum4/2
  Sum4/1 -> System Acc. Efficiency/2
  [ConsumedPower] -> Sum5/1
  Constant9/1 -> Sum5/2
  Sum5/1 -> System inst. Efficiency/2
  IC1/1 -> Divide1/2
  Max/1 -> Transport Delay/1
  Transport Delay/1 -> Simulink-PS Converter2/1
  Transport Delay1/1 -> Simulink-PS Converter1/1
  Divide2/1 -> Transport Delay1/1
  Add1/1 -> If/1
  Initial condition heat storage1/1 -> Add1/1
  [StoredHeatEnergy] -> Add1/2
  If/1 -> If Action Subsystem/Action
  [HeatBalance] -> If Action Subsystem/1(In1)
  If/2 -> If Action Subsystem1/Action
  If Action Subsystem/1(Out1) -> Merge/2
  If Action Subsystem1/1(Out1) -> Merge/1
  Merge/1 -> Heat to storage [W]/1
  Initial condition heat storage2/1 -> System Acc. Efficiency1/2
  Initial condition heat storage/1 -> System Acc. Efficiency1/1
  System Acc. Efficiency1/1 -> Stored heat [J]/2
  Stored heat [J]/1 -> Stored Heat [J]/1
  Initial condition heat storage3/1 -> Divide/2
  [StoredHeatEnergy] -> Divide/1
  Divide/1 -> [HeatStorageSOC]
  [HydrogenCons] -> LH2 ColdRecovery Enthalpy gain/1
  LH2 ColdRecovery Enthalpy gain/1 -> LH2 ColdRecovery Efficiency/1
  LH2 ColdRecovery Efficiency/1 -> [LH2ColdRecovery_Available]
  [CoolDemandPow] -> Subtract/1
  [LH2ColdRecoveredPower] -> Subtract/2
  Subtract/1 -> Cooling Elec Power/1
  [CoolDemandPow] -> Saturation Dynamic/1
  [LH2ColdRecovery_Available] -> Saturation Dynamic/2
  Constant6/1 -> Saturation Dynamic/3
  Saturation Dynamic/1 -> Power to energy3/1, LH2 ColdRecovery Power/1
  [LH2ColdRecoveredPower] -> Add2/5
  Power to energy3/1 -> Energy (MWh)3/1
  Energy (MWh)3/1 -> [LH2ColdRecoveredEnergy]
  connections:
  Voltage Sensor1/RConn1 -- PS-Simulink Converter2/LConn1
  Voltage Sensor1/LConn1 -- Current Sensor/LConn1 -- Controlled Voltage Source/LConn1
  Simulink-PS Converter2/RConn1 -- Controlled Voltage Source/RConn1
  Controlled Voltage Source/RConn2 -- Electrical Reference/LConn1 -- FC-/RConn1 -- Voltage Sensor1/RConn2
  Simulink-PS Converter1/RConn1 -- Duty Cycle/RConn1
  PS-Simulink Converter1/LConn1 -- Current Sensor/RConn1
  FC+/RConn1 -- Current Sensor/RConn2

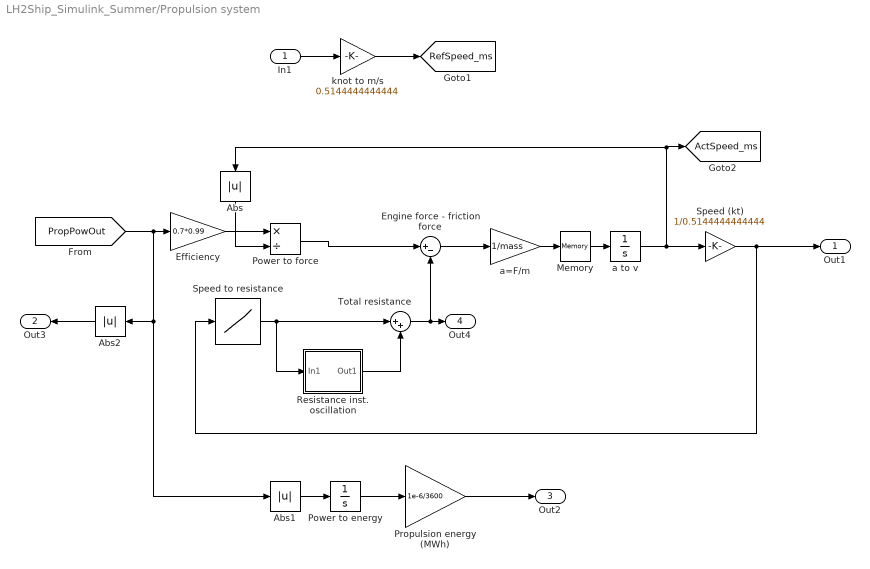
== system LH2Ship_Simulink_Summer/Propulsion system ==
  In1 : Inport
  Abs : Abs  SaturateOnIntegerOverflow=off
  Abs1 : Abs  SaturateOnIntegerOverflow=off
  Abs2 : Abs  SaturateOnIntegerOverflow=off
  Efficiency : Gain  Gain=0.7*0.99
  Engine force - friction force : Sum  Inputs=|+-
  Memory : Memory  InitialCondition=16.66*0.51444444
  Power to energy : Integrator  LowerSaturationLimit=0
  Power to force : Product  Inputs=*/
  Propulsion energy (MWh) : Gain  Gain=1e-6/3600
  Resistance inst. oscillation : Subsystem
  Speed (kt) : Gain  Gain=1/0.5144444444444
  Speed to resistance : Lookup  InputValues=v  Table=Rt  SaturateOnIntegerOverflow=off
  Total resistance : Sum  Inputs=|++
  a to v : Integrator  InitialCondition=16.66*0.51444444  LowerSaturationLimit=0
  a=F/m : Gain  Gain=1/mass
  knot to m/s : Gain  Gain=0.5144444444444
  Out1 : Outport  VectorParamsAs1DForOutWhenUnconnected=off
  Out3 : Outport  Port=2  VectorParamsAs1DForOutWhenUnconnected=off
  Out2 : Outport  Port=3  VectorParamsAs1DForOutWhenUnconnected=off
  Out4 : Outport  Port=4  VectorParamsAs1DForOutWhenUnconnected=off
  tag scope: ActSpeed_ms=global, RefSpeed_ms=global
  wires:
  Speed to resistance/1 -> Resistance inst. oscillation/1(In1), Total resistance/1
  Propulsion energy (MWh)/1 -> Out2/1
  Resistance inst. oscillation/1(Out1) -> Total resistance/2
  a to v/1 -> [ActSpeed_ms], Abs/1, Speed (kt)/1
  Abs/1 -> Power to force/2
  Total resistance/1 -> Out4/1, Engine force - friction force/2
  Power to energy/1 -> Propulsion energy (MWh)/1
  Abs1/1 -> Power to energy/1
  Speed (kt)/1 -> Speed to resistance/1, Out1/1
  [PropPowOut] -> Abs2/1, Abs1/1, Efficiency/1
  In1/1 -> knot to m/s/1
  Power to force/1 -> Engine force - friction force/1
  Engine force - friction force/1 -> a=F/m/1
  Efficiency/1 -> Power to force/1
  a=F/m/1 -> Memory/1
  Memory/1 -> a to v/1
  Abs2/1 -> Out3/1
  knot to m/s/1 -> [RefSpeed_ms]
